simulink model "control_sim"  (R2025a)
settings: Solver=VariableStepAuto  StartTime=0.0  StopTime=10.0  RelTol=1e-3
settings Model: Creator=henri  LastModifiedBy=guilherme-lazzarini

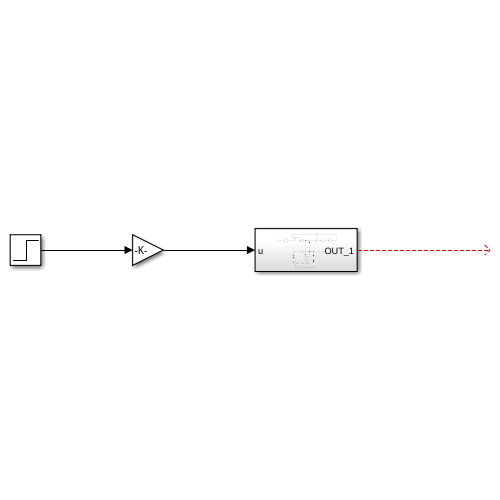
[thumbnail: Simulink's stored preview of the top-level diagram]
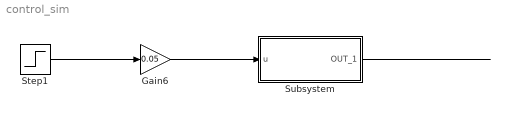
== system control_sim ==
  Gain6 : Gain  Gain=0.05
  Step1 : Step  SampleTime=0
  Subsystem : Subsystem
  wires:
  Step1/1 -> Gain6/1
  Gain6/1 -> Subsystem/1(u)
  Subsystem/1(OUT_1) -> ?

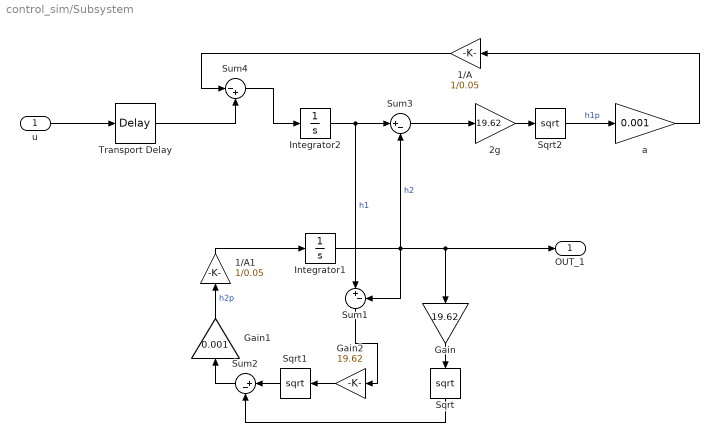
== system control_sim/Subsystem ==
  u : Inport
  1/A : Gain  Gain=1/0.05
  1/A1 : Gain  Gain=1/0.05
  2g : Gain  Gain=19.62
  Gain : Gain  Gain=19.62
  Gain1 : Gain  Gain=0.001
  Gain2 : Gain  Gain=19.62
  Integrator1 : Integrator
  Integrator2 : Integrator
  Sqrt : Sqrt
  Sqrt1 : Sqrt
  Sqrt2 : Sqrt
  Sum1 : Sum  Inputs=|+-
  Sum2 : Sum  Inputs=|+-
  Sum3 : Sum  Inputs=|+-
  Sum4 : Sum  Inputs=|-+
  Transport Delay : TransportDelay  DelayTime=0.005
  a : Gain  Gain=0.001
  OUT_1 : Outport
  wires:
  Sqrt/1 -> Sum2/2
  Sum3/1 -> 2g/1
  2g/1 -> Sqrt2/1
  Gain2/1 -> Sqrt1/1
  Gain/1 -> Sqrt/1
  Integrator1/1 -> Sum3/2, OUT_1/1, Gain/1, Sum1/2  "h2"
  Integrator2/1 -> Sum3/1, Sum1/1  "h1"
  Sum2/1 -> Gain1/1
  Sqrt1/1 -> Sum2/1
  Sqrt2/1 -> a/1  "h1p"
  Sum1/1 -> Gain2/1
  u/1 -> Transport Delay/1
  a/1 -> 1/A/1
  Sum4/1 -> Integrator2/1
  Transport Delay/1 -> Sum4/2
  1/A/1 -> Sum4/1
  1/A1/1 -> Integrator1/1
  Gain1/1 -> 1/A1/1  "h2p"
